simulink model "duffingNL"  (R2020a)
settings: Solver=VariableStepAuto  StartTime=0.0  StopTime=10  RelTol=1e-3
undefined symbols (not defined in the file or in its folder): alpha, duffing_func, g, k, l, m, x_init
libraries: simulink x1
settings Model: Creator=jbrouill  LastModifiedBy=clara
settings OptimizationCC: BlockReduction=off  DefaultParameterBehavior=Inlined  BufferReuse=off

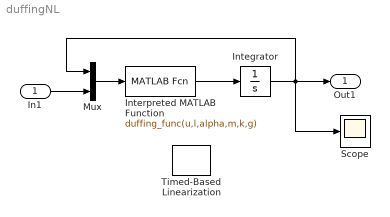
== system duffingNL ==
  In1 : Inport
  Integrator : Integrator  InitialCondition=x_init
  Interpreted MATLAB Function : MATLABFcn  MATLABFcn=duffing_func(u,l,alpha,m,k,g)
  Mux : Mux  Inputs=2
  Scope : Scope
  Timed-Based Linearization : simulink/Model-Wide Utilities/Timed-Based Linearization  LinearizationTime=10  SampleTime=0
      settings: SourceProductBaseCode=SL
  Out1 : Outport
  wires:
  Mux/1 -> Interpreted MATLAB Function/1
  Interpreted MATLAB Function/1 -> Integrator/1
  Integrator/1 -> Scope/1, Out1/1, Mux/1
  In1/1 -> Mux/2
